simulink model "TSMCDTC"  (R2015b)
settings: Solver=VariableStepAuto  StartTime=0.0  StopTime=0.2  RelTol=1e-3
model workspace (MAT data in the model file):
  J = 0.089
  Lm = 0.06931
  Lr = 0.07131
  Ls = 0.07131
  P = 4
  Rr = 0.816
  Rs = 0.435
  theta0 = 0
undefined symbols (not defined in the file or in its folder): magnitude
libraries: powerlib x32, simulink x2
settings Model: PauseTimes=0.0134  Creator=yoush  LastModifiedBy=yoush
settings DataIOCC: SaveFormat=Array
settings DebuggingCC: UnderspecifiedInitializationDetection=Classic  MergeDetectMultiDrivingBlocksExec=none  SolverPrmCheckMsg=warning
settings HardwareCC: ProdBitPerPointer=32  ProdLargestAtomicFloat=None  ProdIntDivRoundTo=Undefined  ProdEndianess=Unspecified  ProdWordSize=32  ProdHWDeviceType=32-bit Generic
settings GRTTargetCC: GeneratePreprocessorConditionals=Disable all
settings ConfigComp: CovModelRefEnable=Off

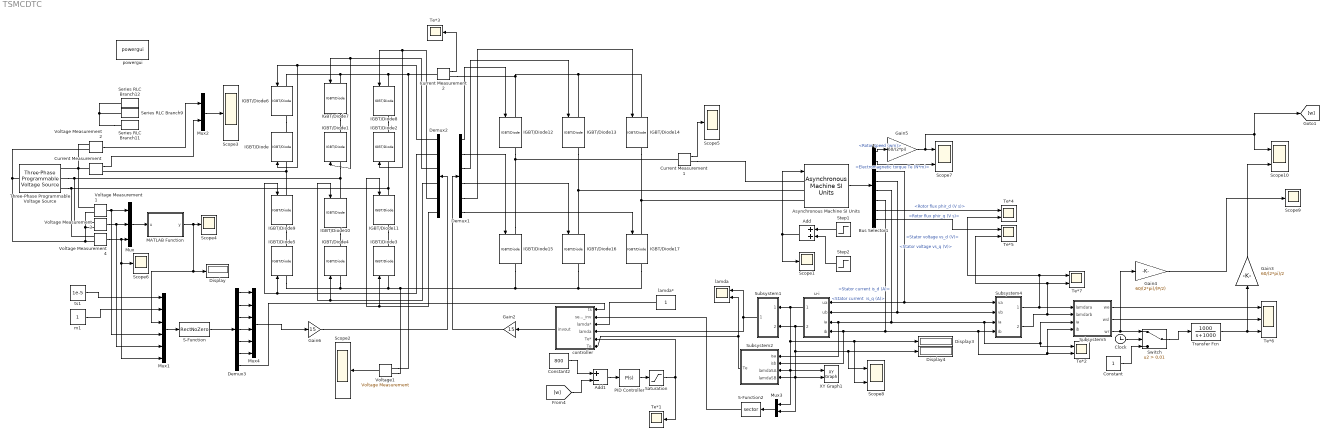
== system TSMCDTC ==
  Add : Sum
  Add1 : Sum  Inputs=+-
  Asynchronous Machine SI Units : powerlib/Machines/Asynchronous Machine SI Units  RotorType=Squirrel-cage  PresetModel=No  MechanicalLoad=Torque Tm  ShowDetailedParameters=on  ReferenceFrame=Stationary  Units=SI  MeasurementBus=off  NominalParameters=[22000 380 50]  Stator=[0.435 2e-3]  Rotor=[0.816 2e-3]  Cage1=[0.4155 0.002066]  Cage2=[0.4168 0.0003495]  Lm=69.31e-3  Mechanical=[0.089 0 2]  PolePairs=2  InitialConditions=[ 1 0 0 0 0 0 0 0]  SimulateSaturation=off  Saturation=[14.03593122, 27.81365428, 53.79336849, 72.68890987, 97.98006896, 148.6815601, 215.7428561, 302.9841135, 428.7778367 ; 230, 322, 414, 460, 506, 552, 598, 644, 690]  LoadFlowParameters=1492000  TsPowergui=0  TsBlock=-1  IterativeModel=Trapezoidal non iterative  Pmec=1.492e+006
  Bus Selector1 : BusSelector  OutputSignals="Mechanical.Rotor speed (wm),Mechanical.Electromagnetic torque Te (N*m),Stator measurements.Stator voltage vs_d (V),Stator measurements.Stator voltage vs_q (V),Stator measurements.Stator current is_d (A),Stator measurements.Stator current  is_q (A),Rotor measurements.Rotor flux phir_d (V s),Rotor measurements.Rotor flux phir_q (V s)"
  Clock : Clock
  Constant : Constant
  Constant2 : Constant  Value=800
  Current Measurement : powerlib/Measurements/Current Measurement  PhasorSimulation=off  OutputType=Complex  PSBequivalent=0
  Current Measurement1 : powerlib/Measurements/Current Measurement  PhasorSimulation=off  OutputType=Complex  PSBequivalent=0
  Current Measurement2 : powerlib/Measurements/Current Measurement  PhasorSimulation=off  OutputType=Complex  PSBequivalent=0
  Demux1 : Demux  Outputs=6
  Demux2 : Demux  Outputs=6
  Demux3 : Demux  Outputs=7
  Display : Display
  Display3 : Display
  Display4 : Display
  Gain2 : Gain  Gain=15
  Gain3 : Gain  Gain=60/(2*pi)/2
  Gain4 : Gain  Gain=60/(2*pi)/(P/2)
  Gain5 : Gain  Gain=60/(2*pi)
  Gain6 : Gain  Gain=15
  IGBT/Diode{,1..17} (18 alike) : powerlib/Power Electronics/IGBT//Diode  Ron=1e-3  Rs=1e5  Cs=inf  Measurements=on
  MATLAB Function : MATLAB Function  TreatAsAtomicUnit=on
  Mux : Mux  Inputs=3
  Mux1 : Mux  Inputs=6
  Mux2 : Mux  Inputs=2
  Mux3 : Mux  Inputs=2
  Mux4 : Mux  Inputs=6
  PID Controller : simulink/Continuous/PID Controller  Controller=P  TimeDomain=Continuous-time  SampleTime=-1  IntegratorMethod=Forward Euler  FilterMethod=Forward Euler  Form=Parallel  UseFilter=on  ControllerParametersSource=internal  P=5  I=0  D=0  N=100  InitialConditionSource=internal  InitialConditionForIntegrator=0  InitialConditionForFilter=0  ExternalReset=none  LimitOutput=off  UpperSaturationLimit=inf  LowerSaturationLimit=-inf  LinearizeAsGain=on  AntiWindupMode=none  Kb=1  TrackingMode=off  Kt=1  PParamMin=[]  PParamMax=[]  IParamMin=[]  IParamMax=[]  DParamMin=[]  DParamMax=[]  NParamMin=[]  NParamMax=[]  KbParamMin=[]  KbParamMax=[]  KtParamMin=[]  KtParamMax=[]  POutMin=[]  POutMax=[]  IOutMin=[]  IOutMax=[]  DOutMin=[]  DOutMax=[]  NOutMin=[]  NOutMax=[]  KbOutMin=[]  KbOutMax=[]  KtOutMin=[]  KtOutMax=[]  IntegratorOutMin=[]  IntegratorOutMax=[]  FilterOutMin=[]  FilterOutMax=[]  SumOutMin=[]  SumOutMax=[]  SumI1OutMin=[]  SumI1OutMax=[]  SumI2OutMin=[]  SumI2OutMax=[]  SumI3OutMin=[]  SumI3OutMax=[]  SumDOutMin=[]  SumDOutMax=[]  SaturationOutMin=[]  SaturationOutMax=[]  IntegratorContinuousStateAttributes=''  IntegratorStateMustResolveToSignalObject=off  IntegratorRTWStateStorageClass=Auto  FilterContinuousStateAttributes=''  FilterStateMustResolveToSignalObject=off  FilterRTWStateStorageClass=Auto  DifferentiatorICPrevScaledInput=0  DifferentiatorOutMin=[]  DifferentiatorOutMax=[]
  S-Function : S-Function  FunctionName=RectNoZero  SFunctionDeploymentMode=off  EnableBusSupport=off
  S-Function2 : S-Function  FunctionName=sector  SFunctionDeploymentMode=off  EnableBusSupport=off
  Saturation : Saturate  UpperLimit=200  LowerLimit=-10
  Scope{1..6,9} (7 alike) : Scope
  Scope10 : Scope  NumInputPorts=2
  Scope7 : Scope  NumInputPorts=2
  Scope8 : Scope  NumInputPorts=2
  Series RLC Branch11 : powerlib/Elements/Series RLC Branch  LConnTagsString=__new0  RConnTagsString=__new0  BranchType=C  Resistance=1  Inductance=0.5e-3  SetiL0=off  InitialCurrent=0  Capacitance=1e-4  Setx0=off  InitialVoltage=0  Measurements=None
  Series RLC Branch12 : powerlib/Elements/Series RLC Branch  LConnTagsString=__new0  RConnTagsString=__new0  BranchType=C  Resistance=1  Inductance=0.5e-3  SetiL0=off  InitialCurrent=0  Capacitance=1e-4  Setx0=off  InitialVoltage=0  Measurements=None
  Series RLC Branch9 : powerlib/Elements/Series RLC Branch  LConnTagsString=__new0  RConnTagsString=__new0  BranchType=C  Resistance=1  Inductance=0.5e-3  SetiL0=off  InitialCurrent=0  Capacitance=1e-4  Setx0=off  InitialVoltage=0  Measurements=None
  Step1 : Step  Time=0.1  After=100  SampleTime=0
  Step2 : Step  Time=0.15  After=50  SampleTime=0
  Subsystem1 : Subsystem
  Subsystem2 : Subsystem
  Subsystem4 : Subsystem
  Subsystem5 : Subsystem
  Switch : Switch  Criteria=u2 > Threshold  Threshold=0.01
  Te*1 : Scope
  Te*{2,4..5,7} (4 alike) : Scope  NumInputPorts=2
  Te*3 : Scope
  Te*6 : Scope  NumInputPorts=3
  Three-Phase Programmable Voltage Source : powerlib/Electrical Sources/Three-Phase Programmable Voltage Source  PositiveSequence="[380  0 50]"  VariationEntity=None  VariationType=Table of time-amplitude pairs  VariationTypeAlt=Step  VariationStep=0.5  VariationRate=10  VariationMagnitude=0.3  VariationFrequency=2  VariationTiming=[1 2]  VariationPhaseA=off  Amplitudes=[1 0.8 1.2 1.0]  TimeValues=[0 0.1 0.15 0.2]  HarmonicGeneration=off  HarmonicA=[3 0.2 -25 0]  HarmonicB=[2 0.15 35 2]  Timing="[0.05  3]"  BusType=swing  Pref=0  Qref=0  Qmin=-inf  Qmax=inf
  Transfer Fcn : TransferFcn  Numerator=[1000]  Denominator=[1 1000]
  Voltage Measurement{1..4} (4 alike) : powerlib/Measurements/Voltage Measurement  PhasorSimulation=off  OutputType=Complex  PSBequivalent=0
  Voltage1 : powerlib/Measurements/Voltage Measurement  PhasorSimulation=off  OutputType=Complex  PSBequivalent=0
  XY Graph1 : simulink/Sinks/XY Graph  xmin=-1.5  xmax=1.5  ymin=-1.5  ymax=1.5  st=-1
  controller : Subsystem
  lamda : Scope  NumInputPorts=2
  lamda* : Constant
  m1 : Constant
  powergui : powerlib/powergui  Priority=1  SimulationMode=Discrete  SolverType=Tustin  SampleTime=1e-6  frequency=60  SPID=off  DisableSnubberDevices=off  DisableRonSwitches=off  DisableVfSwitches=off  SwTol=0  DisplayEquations=off  Interpol=off  ExternalGateDelay=off  methode=off  Ts=0  FunctionMessages=off  echomessages=off  HookPort=off  EnableUseOfTLC=off  x0status=blocks  frequencyindice=50  Pbase=100e6  ErrMax=1e-4  Iterations=50  UnitsV=kV  UnitsW=MW  buscounter=0  RestoreLinks=warning  ResistiveCurrentMeasurement=off  Frange=[0:2:500]  Ylog=off  Xlog=on  ShowGrid=off  save=off  variable=ZData  structure=wr  ZoomFFT=off  StartTime=0.16  cycles=2  DisplayStyle=2  fundamental=100  FreqAxis=off  MaxFrequency=10000  frequencyindicesteady=1  RmsSteady=1  display=off
  ts1 : Constant  Value=1e-5
  u-i : Subsystem
  wires:
  Mux2/1 -> Scope3/1
  Demux2/1 -> IGBT/Diode/1, IGBT/Diode6/1
  Demux2/3 -> IGBT/Diode1/1, IGBT/Diode7/1
  Demux2/5 -> IGBT/Diode2/1, IGBT/Diode8/1
  Demux2/2 -> IGBT/Diode9/1, IGBT/Diode5/1
  Demux2/4 -> IGBT/Diode10/1, IGBT/Diode4/1
  Demux2/6 -> IGBT/Diode11/1, IGBT/Diode3/1
  Demux1/1 -> IGBT/Diode12/1
  Demux1/3 -> IGBT/Diode13/1
  Demux1/5 -> IGBT/Diode14/1
  Demux1/2 -> IGBT/Diode15/1
  Demux1/4 -> IGBT/Diode16/1
  Demux1/6 -> IGBT/Diode17/1
  Voltage Measurement2/1 -> Mux2/1
  Current Measurement1/1 -> Scope5/1
  Voltage Measurement1/1 -> Mux/1, Mux1/4
  Voltage Measurement3/1 -> Mux/2, Mux1/5
  Voltage Measurement4/1 -> Scope6/1, Mux1/6, Mux/3
  Mux/1 -> MATLAB Function/1(u)
  MATLAB Function/1(y) -> Display/1, Mux1/3, Scope4/1
  m1/1 -> Mux1/2
  ts1/1 -> Mux1/1
  Mux1/1 -> S-Function/1
  Current Measurement/1 -> Mux2/2
  Asynchronous Machine SI Units/1 -> Bus Selector1/1
  Bus Selector1/2 -> Scope7/2  "<Electromagnetic torque Te (N*m)>"
  Bus Selector1/1 -> Gain5/1  "<Rotor speed (wm)>"
  Bus Selector1/3 -> u-i/1(ua), Subsystem4/1(va)  "<Stator voltage vs_d (V)>"
  Bus Selector1/4 -> Subsystem4/2(vb), u-i/2(ub)  "<Stator voltage vs_q (V)>"
  Bus Selector1/5 -> Te*2/1, Subsystem5/3(ia), Subsystem4/3(ia), Subsystem2/1(isa), u-i/3(ia)  "<Stator current is_d (A)>"
  Bus Selector1/6 -> Subsystem2/2(isb), u-i/4(ib), Te*2/2, Subsystem5/4(ib), Subsystem4/4(ib)  "<Stator current  is_q (A)>"
  Subsystem4/1(lamdara) -> Te*4/2, Te*7/1, Subsystem5/1(lamdara)
  Subsystem4/2(lamdarb) -> Te*7/2, Te*5/2, Subsystem5/2(lamdarb)
  Subsystem5/2(wsl) -> Te*6/2
  Subsystem5/3(wr) -> Switch/1, Gain4/1
  u-i/2(lamdaSB) -> Scope8/1, Display4/1, Mux3/2, XY Graph1/2, Subsystem2/4(lamdaSB), Subsystem1/2(beta)
  u-i/1(lamdaSA) -> Scope8/2, Display3/1, Mux3/1, Subsystem2/3(lamdaSA), XY Graph1/1, Subsystem1/1(alpha)
  Step1/1 -> Add/1
  Step2/1 -> Add/2
  Add/1 -> Asynchronous Machine SI Units/1, Scope1/1
  Subsystem1/1(total) -> controller/4(lamda), lamda/1
  Subsystem2/1(Te) -> controller/6(Te), lamda/2
  Mux3/1 -> S-Function2/1
  PID Controller/1 -> Saturation/1
  Add1/1 -> PID Controller/1
  Constant2/1 -> Add1/1
  [w] -> Add1/2
  Saturation/1 -> Te*1/1, controller/5(Te*)
  lamda*/1 -> controller/3(lamda*)
  Voltage1/1 -> Scope2/1
  S-Function2/1 -> controller/2(sector_inv)
  Gain2/1 -> Demux1/1
  Gain6/1 -> Demux2/1
  Current Measurement2/1 -> Te*3/1
  Gain4/1 -> Scope9/1
  Subsystem5/1(we) -> Te*6/1
  controller/1(invout) -> Gain2/1
  S-Function/1 -> Demux3/1
  Demux3/1 -> Mux4/1
  Demux3/2 -> Mux4/2
  Demux3/3 -> Mux4/3
  Demux3/4 -> Mux4/4
  Demux3/5 -> Mux4/5
  Demux3/6 -> Mux4/6
  Mux4/1 -> Gain6/1
  Demux3/7 -> controller/1(ts)
  Transfer Fcn/1 -> Gain3/1, Te*6/3
  Switch/1 -> Transfer Fcn/1
  Constant/1 -> Switch/3
  Clock/1 -> Switch/2
  Bus Selector1/7 -> Te*4/1  "<Rotor flux phir_d (V s)>"
  Bus Selector1/8 -> Te*5/1  "<Rotor flux phir_q (V s)>"
  Gain5/1 -> Scope10/1, [w], Scope7/1
  Gain3/1 -> Scope10/2
  connections:
  Three-Phase Programmable Voltage Source/RConn2 -- IGBT/Diode1/LConn1 -- IGBT/Diode10/LConn1 -- Voltage Measurement3/LConn1
  Three-Phase Programmable Voltage Source/RConn3 -- IGBT/Diode11/LConn1 -- IGBT/Diode2/LConn1 -- Voltage Measurement4/LConn1
  IGBT/Diode10/RConn1 -- IGBT/Diode4/RConn1
  IGBT/Diode9/RConn1 -- IGBT/Diode5/RConn1
  Series RLC Branch11/LConn1 -- Series RLC Branch12/LConn1 -- Series RLC Branch9/LConn1
  IGBT/Diode6/RConn1 -- IGBT/Diode/RConn1
  IGBT/Diode11/RConn1 -- IGBT/Diode3/RConn1
  IGBT/Diode8/RConn1 -- IGBT/Diode2/RConn1
  IGBT/Diode7/RConn1 -- IGBT/Diode1/RConn1
  IGBT/Diode15/LConn1 -- IGBT/Diode12/RConn1 -- Current Measurement1/LConn1
  Voltage Measurement2/LConn1 -- Voltage Measurement1/LConn1 -- Three-Phase Programmable Voltage Source/RConn1 -- Current Measurement/LConn1
  Voltage Measurement2/LConn2 -- Voltage Measurement1/LConn2 -- Voltage Measurement3/LConn2 -- Voltage Measurement4/LConn2 -- Three-Phase Programmable Voltage Source/LConn1
  IGBT/Diode13/RConn1 -- Asynchronous Machine SI Units/LConn2 -- IGBT/Diode16/LConn1
  IGBT/Diode14/RConn1 -- IGBT/Diode17/LConn1 -- Asynchronous Machine SI Units/LConn3
  IGBT/Diode7/LConn1 -- IGBT/Diode6/LConn1 -- Current Measurement2/LConn1 -- Voltage1/LConn1 -- IGBT/Diode8/LConn1
  IGBT/Diode17/RConn1 -- IGBT/Diode16/RConn1 -- IGBT/Diode5/LConn1 -- IGBT/Diode4/LConn1 -- IGBT/Diode3/LConn1 -- Voltage1/LConn2 -- IGBT/Diode15/RConn1
  IGBT/Diode12/LConn1 -- Current Measurement2/RConn1 -- IGBT/Diode13/LConn1 -- IGBT/Diode14/LConn1
  Current Measurement1/RConn1 -- Asynchronous Machine SI Units/LConn1
  IGBT/Diode9/LConn1 -- Current Measurement/RConn1 -- IGBT/Diode/LConn1

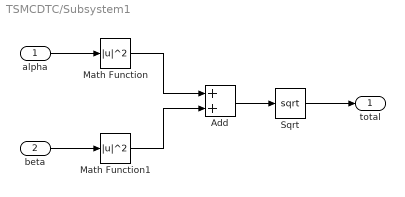
== system TSMCDTC/Subsystem1 ==
  alpha : Inport
  beta : Inport  Port=2
  Add : Sum
  Math Function : Math  Operator=magnitude^2  SaturateOnIntegerOverflow=on
  Math Function1 : Math  Operator=magnitude^2  SaturateOnIntegerOverflow=on
  Sqrt : Sqrt  SaturateOnIntegerOverflow=on
  total : Outport
  wires:
  alpha/1 -> Math Function/1
  beta/1 -> Math Function1/1
  Math Function/1 -> Add/1
  Math Function1/1 -> Add/2
  Add/1 -> Sqrt/1
  Sqrt/1 -> total/1

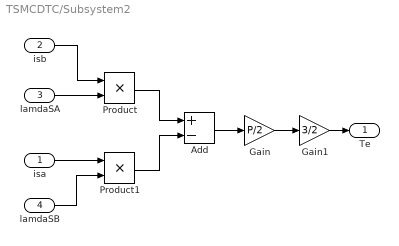
== system TSMCDTC/Subsystem2 ==
  isa : Inport
  isb : Inport  Port=2
  lamdaSA : Inport  Port=3
  lamdaSB : Inport  Port=4
  Add : Sum  Inputs=+-
  Gain : Gain  Gain=P/2
  Gain1 : Gain  Gain=3/2
  Product : Product
  Product1 : Product
  Te : Outport
  wires:
  Add/1 -> Gain/1
  Product/1 -> Add/1
  Product1/1 -> Add/2
  lamdaSA/1 -> Product/2
  isb/1 -> Product/1
  isa/1 -> Product1/1
  lamdaSB/1 -> Product1/2
  Gain/1 -> Gain1/1
  Gain1/1 -> Te/1

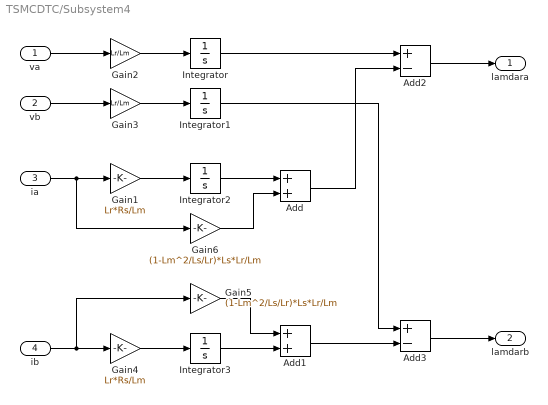
== system TSMCDTC/Subsystem4 ==
  va : Inport
  vb : Inport  Port=2
  ia : Inport  Port=3
  ib : Inport  Port=4
  Add : Sum
  Add1 : Sum
  Add2 : Sum  Inputs=+-
  Add3 : Sum  Inputs=+-
  Gain1 : Gain  Gain=Lr*Rs/Lm
  Gain2 : Gain  Gain=Lr/Lm
  Gain3 : Gain  Gain=Lr/Lm
  Gain4 : Gain  Gain=Lr*Rs/Lm
  Gain5 : Gain  Gain=(1-Lm^2/Ls/Lr)*Ls*Lr/Lm
  Gain6 : Gain  Gain=(1-Lm^2/Ls/Lr)*Ls*Lr/Lm
  Integrator{,1..3} (4 alike) : Integrator
  lamdara : Outport
  lamdarb : Outport  Port=2
  wires:
  va/1 -> Gain2/1
  Gain2/1 -> Integrator/1
  vb/1 -> Gain3/1
  Gain3/1 -> Integrator1/1
  ia/1 -> Gain6/1, Gain1/1
  Gain1/1 -> Integrator2/1
  ib/1 -> Gain5/1, Gain4/1
  Gain4/1 -> Integrator3/1
  Integrator2/1 -> Add/1
  Gain6/1 -> Add/2
  Integrator3/1 -> Add1/2
  Gain5/1 -> Add1/1
  Integrator/1 -> Add2/1
  Add/1 -> Add2/2
  Add2/1 -> lamdara/1
  Add1/1 -> Add3/2
  Integrator1/1 -> Add3/1
  Add3/1 -> lamdarb/1

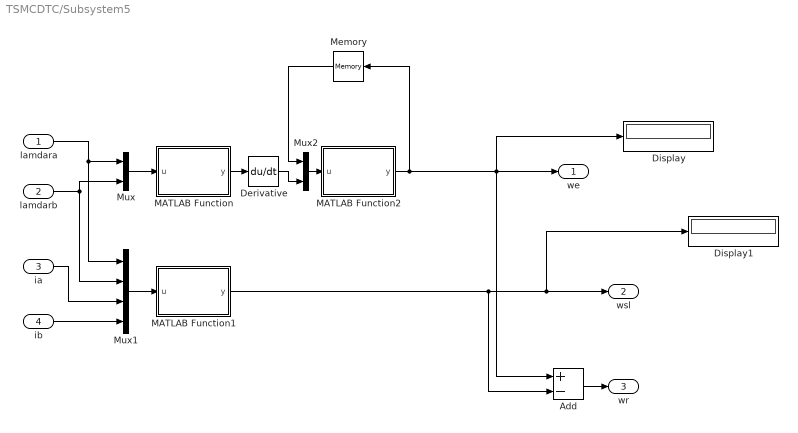
== system TSMCDTC/Subsystem5 ==
  lamdara : Inport
  lamdarb : Inport  Port=2
  ia : Inport  Port=3
  ib : Inport  Port=4
  Add : Sum  Inputs=+-
  Derivative : Derivative
  Display : Display
  Display1 : Display
  MATLAB Function : MATLAB Function  TreatAsAtomicUnit=on
  MATLAB Function1 : MATLAB Function  TreatAsAtomicUnit=on
  MATLAB Function2 : MATLAB Function  TreatAsAtomicUnit=on
  Memory : Memory
  Mux : Mux  Inputs=2
  Mux1 : Mux
  Mux2 : Mux  Inputs=2
  we : Outport
  wsl : Outport  Port=2
  wr : Outport  Port=3
  wires:
  Mux/1 -> MATLAB Function/1(u)
  lamdara/1 -> Mux/1, Mux1/1
  lamdarb/1 -> Mux1/2, Mux/2
  MATLAB Function/1(y) -> Derivative/1
  Mux1/1 -> MATLAB Function1/1(u)
  ia/1 -> Mux1/3
  ib/1 -> Mux1/4
  Add/1 -> wr/1
  MATLAB Function2/1(y) -> Add/1, Display/1, we/1, Memory/1
  MATLAB Function1/1(y) -> Add/2, Display1/1, wsl/1
  Mux2/1 -> MATLAB Function2/1(u)
  Derivative/1 -> Mux2/2
  Memory/1 -> Mux2/1

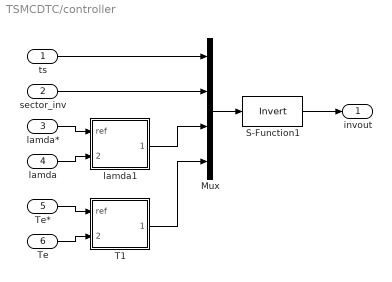
== system TSMCDTC/controller ==
  ts : Inport
  sector_inv : Inport  Port=2
  lamda* : Inport  Port=3
  lamda : Inport  Port=4
  Te* : Inport  Port=5
  Te : Inport  Port=6
  Mux : Mux
  S-Function1 : S-Function  FunctionName=Invert  SFunctionDeploymentMode=off  EnableBusSupport=off
  T1 : Subsystem
  lamda1 : Subsystem
  invout : Outport
  wires:
  Te*/1 -> T1/1(ref)
  Te/1 -> T1/2(measure)
  lamda*/1 -> lamda1/1(ref)
  lamda/1 -> lamda1/2(measure)
  S-Function1/1 -> invout/1
  Mux/1 -> S-Function1/1
  ts/1 -> Mux/1
  sector_inv/1 -> Mux/2
  lamda1/1(Out1) -> Mux/3
  T1/1(Out1) -> Mux/4

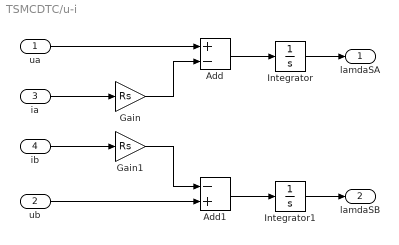
== system TSMCDTC/u-i ==
  ua : Inport
  ub : Inport  Port=2
  ia : Inport  Port=3
  ib : Inport  Port=4
  Add : Sum  Inputs=+-
  Add1 : Sum  Inputs=-+
  Gain : Gain  Gain=Rs
  Gain1 : Gain  Gain=Rs
  Integrator : Integrator
  Integrator1 : Integrator
  lamdaSA : Outport
  lamdaSB : Outport  Port=2
  wires:
  ib/1 -> Gain1/1
  ia/1 -> Gain/1
  Gain/1 -> Add/2
  ua/1 -> Add/1
  ub/1 -> Add1/2
  Gain1/1 -> Add1/1
  Add/1 -> Integrator/1
  Add1/1 -> Integrator1/1
  Integrator1/1 -> lamdaSB/1
  Integrator/1 -> lamdaSA/1

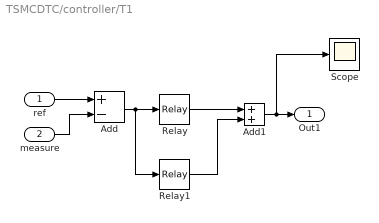
== system TSMCDTC/controller/T1 ==
  ref : Inport
  measure : Inport  Port=2
  Add : Sum  Inputs=+-
  Add1 : Sum
  Relay : Relay  OnSwitchValue=10  OffSwitchValue=-10  OnOutputValue=0.5  OffOutputValue=-0.5
  Relay1 : Relay  OnSwitchValue=0  OffSwitchValue=0  OnOutputValue=0.5  OffOutputValue=-0.5
  Scope : Scope
  Out1 : Outport
  wires:
  Add/1 -> Relay1/1, Relay/1
  ref/1 -> Add/1
  measure/1 -> Add/2
  Relay1/1 -> Add1/2
  Add1/1 -> Scope/1, Out1/1
  Relay/1 -> Add1/1

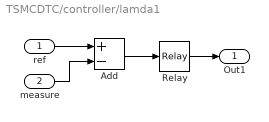
== system TSMCDTC/controller/lamda1 ==
  ref : Inport
  measure : Inport  Port=2
  Add : Sum  Inputs=+-
  Relay : Relay  OnSwitchValue=0.005  OffSwitchValue=-0.005
  Out1 : Outport
  wires:
  Relay/1 -> Out1/1
  Add/1 -> Relay/1
  ref/1 -> Add/1
  measure/1 -> Add/2

== matlab function TSMCDTC/MATLAB Function ==
  data: u input; y output
function y = fcn(u)
if (u(1) > 0 && u(2) < 0 && u(3) <= 0)
    y = 1;
elseif (u(1) > 0 && u(2) >= 0 && u(3) < 0)
    y = 2;
elseif (u(1) <= 0 && u(2) > 0 && u(3) < 0)
    y = 3;
elseif (u(1) < 0 && u(2) > 0 && u(3) >= 0)
    y = 4;
elseif (u(1) < 0 && u(2) <= 0 && u(3) > 0)
    y = 5;
else
    y = 6;
end

== matlab function TSMCDTC/Subsystem5/MATLAB Function ==
  data: u input; y output
function y = fcn(u)
if (u(1) ~= 0)
    y = atan(u(2) / u(1));
else
    y = 0.5 * pi;
end

== matlab function TSMCDTC/Subsystem5/MATLAB Function1 ==
  data: u input; y output
function y = fcn(u)
Lm = 0.06931;
Tr = 0.07131/0.816;

y = Lm/Tr * abs(u(1)*u(4) - u(2)*u(3)) / (u(1)^2 + u(2)^2);

== matlab function TSMCDTC/Subsystem5/MATLAB Function2 ==
  data: u input; y output
function y = fcn(u)
if (abs(u(2)) > 500)
    y = u(1);
else
    y = u(2);
end
